simulink library "libbha_kinematic_tools"  (R2015b)
settings: Solver=FixedStepDiscrete  StartTime=0.0  StopTime=Inf  FixedStep=0.004  RelTol=1e-3
PostLoadFcn:
  | , if any(exist('dsrtsu_mdlpostloadfcn', 'file') == [2, 3, 6]), try dsrtsu_mdlpostloadfcn('Execute', bdroot); catch fprintf('Error in PostLoadFcn (dsrtsu_mdlpostloadfcn) for model "%s":\n %s\n', bdroot, lasterr); end, end,
undefined symbols (not defined in the file or in its folder): BHA
settings Model: DSRTSU_INTERNAL_RTI_VER=440  DSRTSU_INTERNAL_RTI_TYPE=rti1005  DSRTSU_INTERNAL_RTIFPGA=30  Creator=Falkenhahn  LastModifiedBy=Mayer
settings DataIOCC: SaveFormat=Array
settings OptimizationCC: BlockReduction=off  OptimizeBlockIOStorage=off  BufferReuse=off  GlobalBufferReuse=off  ExpressionFolding=off  LocalBlockOutputs=off
settings DebuggingCC: UnderspecifiedInitializationDetection=Classic  MergeDetectMultiDrivingBlocksExec=none  SolverPrmCheckMsg=warning
settings HardwareCC: ProdBitPerPointer=32  ProdLargestAtomicFloat=None  ProdEndianess=BigEndian  ProdWordSize=32  ProdHWDeviceType=Generic->Custom  TargetIntDivRoundTo=Zero  TargetEndianess=BigEndian  TargetHWDeviceType=Generic->Custom
settings RTWCC: SystemTargetFile=rti1007.tlc  MakeCommand=make_rti  TemplateMakefile=rti1007.tmf  Description=dSPACE DS1007 Hardware Platform
settings STFCustomTargetCC: ParMdlRefBuildCompliant=on  ConcurrentExecutionCompliant=off  MatFileLogging=on  SystemTargetFile=rti1007.tlc
settings GRTTargetCC: CompOptLevelCompliant=off  ConcurrentExecutionCompliant=off  GeneratePreprocessorConditionals=Disable all  CombineOutputUpdateFcns=off  GRTInterface=on  UseToolchainInfoCompliant=off  ExtModeMexFile=noextcomm
settings ConfigComp: CovModelRefEnable=Off

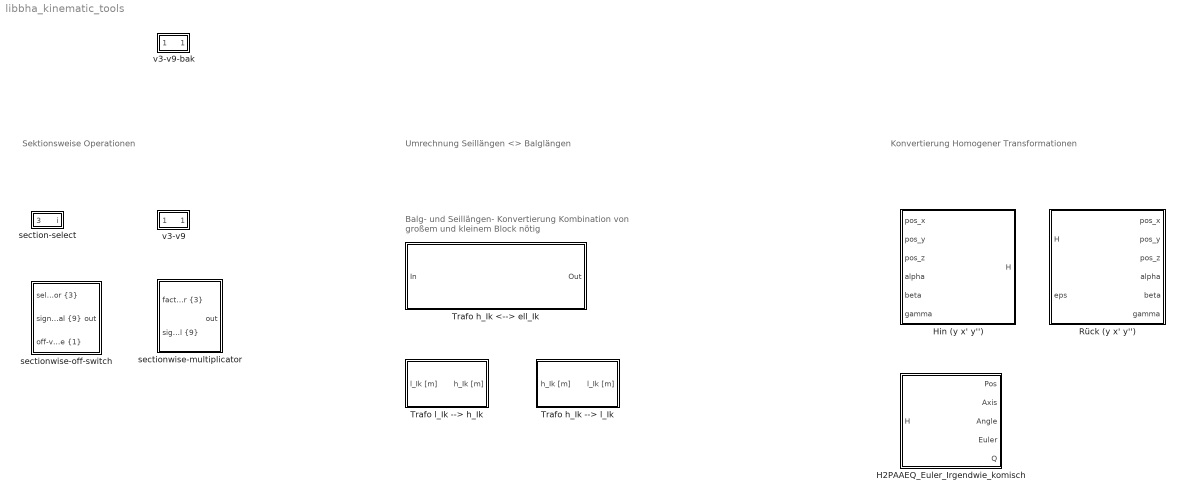
== system libbha_kinematic_tools ==
  note: Balg- und Seillängen- Konvertierung
      | Kombination von großem und kleinem Block nötig
  note: Konvertierung
      | Homogener Transformationen
  note: Umrechnung
      | Seillängen <> Balglängen
  note: Sektionsweise
      | Operationen
  H2PAAEQ_Euler_Irgendwie_komisch : MATLAB Function  TreatAsAtomicUnit=on
  Hin (y x' y'') : MATLAB Function  TreatAsAtomicUnit=on
  Rück (y x' y'') : MATLAB Function  TreatAsAtomicUnit=on
  Trafo h_Ik --> l_Ik : Subsystem  mask{ii=1 = gross}
      mask prompts: ii "Sektionsindex (ii)"
      settings: AttributesFormatString=Seilzughöhe > Seilzuglänge\nSektion = %<ii>
      mask TypeOptions ii: 1 = gross | 2 = mittel | 3 = klein
  Trafo h_Ik <--> ell_Ik : Subsystem  mask{inv=off, ii=1, m_i=BHA.Trunk.vc.num_segm, r_Si=BHA.Trunk.r_ms_i, r_Ai=BHA.Trunk.r_mb_i}
      mask prompts: inv "Transformationsrichtung (inv)"; ii "Sektionsindex (ii)"; m_i "Anzahl der Seilführungen, Segmente (m_i)"; r_Si "Radiale Abstände der Seilzugführungen von der Sektionsbiegelinie der i Sektionen (r_Si)"; r_Ai "Radiale Abstände der Aktoren von der Sektionsbiegelinie der i Sektionen (r_Ai)"
      mask help:
      | Berechnung der Hin- und Rücktransformation:
      | Balgbogenlänge ell_Ik <--> Seilzuglängen h_Ik
      |
      | Transformationsrichtung:
      |     - inv = disable:    h_Ik   --> ell_ik
      |     - inv = enable:     ell_Ik --> h_ik
      settings: AttributesFormatString=Seilzughöhe <> Balgbogenlänge\ninv = %<inv> | Sektion %<ii>
      mask Display: fprintf('inv = disable\n h_Ik -> ell_Ik \n\n inv = enable\n ell_Ik -> h_Ik')
  Trafo l_Ik --> h_Ik : Subsystem  mask{ii=1 = gross}
      mask prompts: ii "Sektionsindex (ii)"
      settings: AttributesFormatString=Seilzuglänge > Seilzughöhe\nSektion %<ii>
      mask TypeOptions ii: 1 = gross | 2 = mittel | 3 = klein
  section-select : Subsystem  mask(Sektionsauswahl){ii=1}
      mask prompts: ii "Sektion"
      mask help: wählt aus einem Parametersatz (Tripple) den der jew. Sektion aus
      settings: AttributesFormatString="in: 3  out: 1"
      mask Display: fprintf('S:%i',ii)
  sectionwise-multiplicator : Subsystem
  sectionwise-off-switch : Subsystem
  v3-v9 : Subsystem
  v3-v9-bak : Subsystem

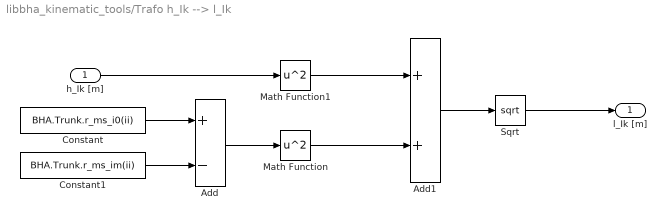
== system libbha_kinematic_tools/Trafo h_Ik --> l_Ik ==
  h_Ik [m] : Inport  PortDimensions=3
  Add : Sum  Inputs=+-
  Add1 : Sum
  Constant : Constant  Value=BHA.Trunk.r_ms_i0(ii)
  Constant1 : Constant  Value=BHA.Trunk.r_ms_im(ii)
  Math Function : Math  Operator=square  SaturateOnIntegerOverflow=on
  Math Function1 : Math  Operator=square  SaturateOnIntegerOverflow=on
  Sqrt : Sqrt  SaturateOnIntegerOverflow=on
  l_Ik [m] : Outport  PortDimensions=3
  wires:
  Constant/1 -> Add/1
  Constant1/1 -> Add/2
  Add/1 -> Math Function/1
  Math Function/1 -> Add1/2
  h_Ik [m]/1 -> Math Function1/1
  Math Function1/1 -> Add1/1
  Add1/1 -> Sqrt/1
  Sqrt/1 -> l_Ik [m]/1

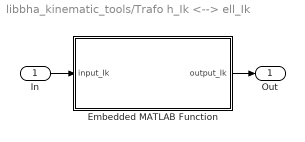
== system libbha_kinematic_tools/Trafo h_Ik <--> ell_Ik ==
  In : Inport  PortDimensions=[3,1]
  Embedded MATLAB Function : MATLAB Function  TreatAsAtomicUnit=on
  Out : Outport  PortDimensions=[3,1]
  wires:
  In/1 -> Embedded MATLAB Function/1(input_Ik)
  Embedded MATLAB Function/1(output_Ik) -> Out/1

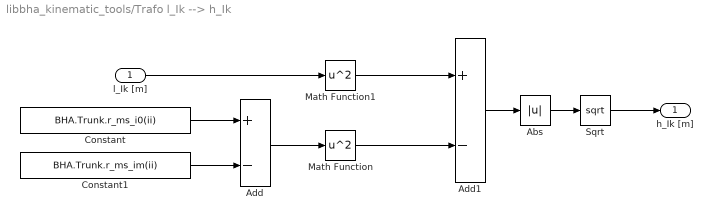
== system libbha_kinematic_tools/Trafo l_Ik --> h_Ik ==
  l_Ik [m] : Inport  PortDimensions=3
  Abs : Abs
  Add : Sum  Inputs=+-
  Add1 : Sum  Inputs=+-
  Constant : Constant  Value=BHA.Trunk.r_ms_i0(ii)
  Constant1 : Constant  Value=BHA.Trunk.r_ms_im(ii)
  Math Function : Math  Operator=square  SaturateOnIntegerOverflow=on
  Math Function1 : Math  Operator=square  SaturateOnIntegerOverflow=on
  Sqrt : Sqrt  SaturateOnIntegerOverflow=on
  h_Ik [m] : Outport  PortDimensions=3
  wires:
  Abs/1 -> Sqrt/1
  Sqrt/1 -> h_Ik [m]/1
  Add1/1 -> Abs/1
  Math Function1/1 -> Add1/1
  l_Ik [m]/1 -> Math Function1/1
  Math Function/1 -> Add1/2
  Add/1 -> Math Function/1
  Constant1/1 -> Add/2
  Constant/1 -> Add/1

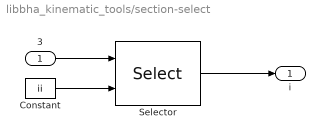
== system libbha_kinematic_tools/section-select ==
  3 : Inport
  Constant : Constant  Value=ii
  Selector : Selector  InputPortWidth=3  IndexOptions=Index vector (port)  Indices=[1 3]  OutputSizes=1
  i : Outport
  wires:
  3/1 -> Selector/1
  Selector/1 -> i/1
  Constant/1 -> Selector/2

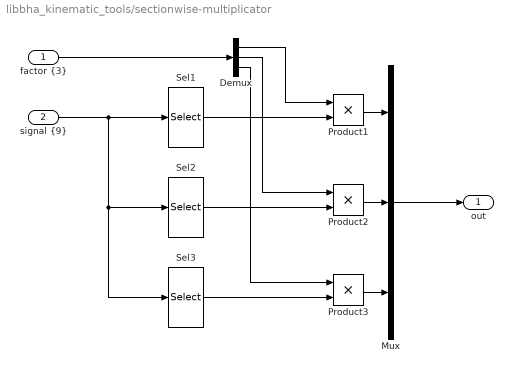
== system libbha_kinematic_tools/sectionwise-multiplicator ==
  "factor {3}" : Inport
  "signal {9}" : Inport  Port=2
  Demux : Demux  Outputs=3
  Mux : Mux  Inputs=3
  Product1 : Product  RndMeth=Zero
  Product2 : Product  RndMeth=Zero
  Product3 : Product  RndMeth=Zero
  Sel1 : Selector  InputPortWidth=9  IndexOptions=Index vector (dialog)  Indices=[1 2 3]  OutputSizes=1
  Sel2 : Selector  InputPortWidth=9  IndexOptions=Index vector (dialog)  Indices=[4 5 6]  OutputSizes=1
  Sel3 : Selector  InputPortWidth=9  IndexOptions=Index vector (dialog)  Indices=[7 8 9]  OutputSizes=1
  out : Outport
  wires:
  Demux/3 -> Product3/1
  Demux/2 -> Product2/1
  Demux/1 -> Product1/1
  Sel1/1 -> Product1/2
  Mux/1 -> out/1
  "signal {9}"/1 -> Sel3/1, Sel2/1, Sel1/1
  Product2/1 -> Mux/2
  Product3/1 -> Mux/3
  Sel3/1 -> Product3/2
  Product1/1 -> Mux/1
  Sel2/1 -> Product2/2
  "factor {3}"/1 -> Demux/1

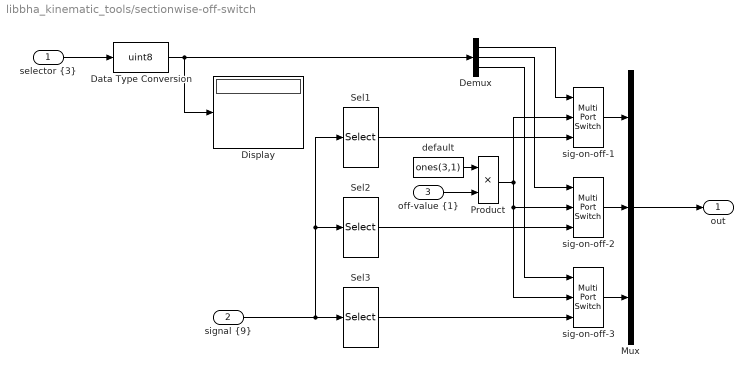
== system libbha_kinematic_tools/sectionwise-off-switch ==
  "selector {3}" : Inport
  "signal {9}" : Inport  Port=2
  "off-value {1}" : Inport  Port=3
  Data Type Conversion : DataTypeConversion  OutDataTypeStr=uint8
  Demux : Demux  Outputs=3
  Display : Display
  Mux : Mux  Inputs=3
  Product : Product  RndMeth=Zero
  Sel1 : Selector  InputPortWidth=9  IndexOptions=Index vector (dialog)  Indices=[1 2 3]  OutputSizes=1
  Sel2 : Selector  InputPortWidth=9  IndexOptions=Index vector (dialog)  Indices=[4 5 6]  OutputSizes=1
  Sel3 : Selector  InputPortWidth=9  IndexOptions=Index vector (dialog)  Indices=[7 8 9]  OutputSizes=1
  default : Constant  Value=ones(3,1)
  sig-on-off-1 : MultiPortSwitch  DataPortOrder=Zero-based contiguous  Inputs=2  DiagnosticForDefault=None
  sig-on-off-2 : MultiPortSwitch  DataPortOrder=Zero-based contiguous  Inputs=2  DiagnosticForDefault=None
  sig-on-off-3 : MultiPortSwitch  DataPortOrder=Zero-based contiguous  Inputs=2  DiagnosticForDefault=None
  out : Outport
  wires:
  Sel1/1 -> sig-on-off-1/3
  Sel2/1 -> sig-on-off-2/3
  Sel3/1 -> sig-on-off-3/3
  Data Type Conversion/1 -> Demux/1, Display/1
  default/1 -> Product/1
  "off-value {1}"/1 -> Product/2
  Demux/3 -> sig-on-off-3/1
  Demux/2 -> sig-on-off-2/1
  Product/1 -> sig-on-off-2/2, sig-on-off-3/2, sig-on-off-1/2
  Demux/1 -> sig-on-off-1/1
  "selector {3}"/1 -> Data Type Conversion/1
  sig-on-off-1/1 -> Mux/1
  sig-on-off-3/1 -> Mux/3
  sig-on-off-2/1 -> Mux/2
  "signal {9}"/1 -> Sel3/1, Sel2/1, Sel1/1
  Mux/1 -> out/1

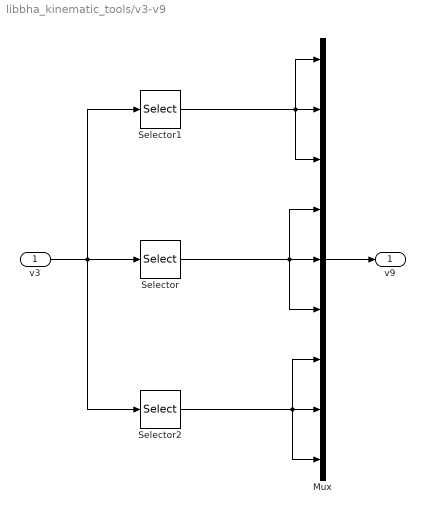
== system libbha_kinematic_tools/v3-v9 ==
  v3 : Inport
  Mux : Mux  Inputs=9
  Selector : Selector  InputPortWidth=3  IndexOptions=Index vector (dialog)  Indices=[2]  OutputSizes=1
  Selector1 : Selector  InputPortWidth=3  IndexOptions=Index vector (dialog)  Indices=[1 ]  OutputSizes=1
  Selector2 : Selector  InputPortWidth=3  IndexOptions=Index vector (dialog)  Indices=[3]  OutputSizes=1
  v9 : Outport
  wires:
  Selector/1 -> Mux/6, Mux/4, Mux/5
  Selector1/1 -> Mux/3, Mux/1, Mux/2
  Selector2/1 -> Mux/9, Mux/7, Mux/8
  Mux/1 -> v9/1
  v3/1 -> Selector2/1, Selector1/1, Selector/1

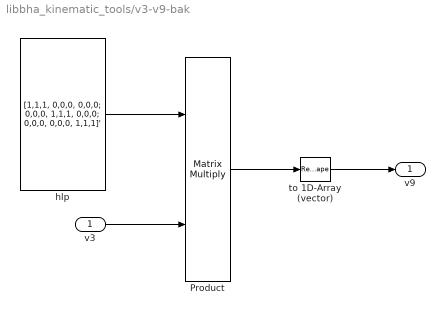
== system libbha_kinematic_tools/v3-v9-bak ==
  v3 : Inport
  Product : Product  Multiplication=Matrix(*)  RndMeth=Zero
  hlp : Constant  Value=[1,1,1, 0,0,0, 0,0,0; 0,0,0, 1,1,1, 0,0,0; 0,0,0, 0,0,0, 1,1,1]'
  to 1D-Array (vector) : Reshape
  v9 : Outport
  wires:
  v3/1 -> Product/2
  hlp/1 -> Product/1
  Product/1 -> to 1D-Array (vector)/1
  to 1D-Array (vector)/1 -> v9/1

== matlab function libbha_kinematic_tools/Hin (y x' y'') ==
  data: pos_x input; pos_y input; pos_z input; alpha input; H output; beta input; gamma input
function H = EulerYXY2H(pos_x, pos_y, pos_z, alpha, beta, gamma)
%#codegen

%H = [   cos(beta)*cos(gamma)    cos(alpha)*sin(gamma)+sin(alpha)*sin(beta)*cos(gamma)   sin(alpha)*sin(gamma)-cos(alpha)*sin(beta)*cos(gamma)   2; ...
%        -cos(beta)*sin(gamma)   cos(alpha)*cos(gamma)-sin(alpha)*sin(beta)*sin(gamma)   sin(alpha)*cos(gamma)+cos(alpha)*sin(beta)*sin(gamma)   3; ...
%        sin(beta)               -sin(alpha)*cos(beta)                                   cos(alpha)*cos(beta)                                    4; ...
%        0                                                       0                                                       0                       1 ];

% Drehung um y
A1 = [  cos(alpha)  0   sin(alpha)  ;
        0           1   0           ;
        -sin(alpha) 0   cos(alpha)  ];


% Drehung um x
A2 = [  1   0           0           ;
        0   cos(beta)   -sin(beta)  ;
        0   sin(beta)   cos(beta)   ];

% Drehung um y
A3 = [  cos(gamma)  0   sin(gamma)  ;
        0           1   0           ;
        -sin(gamma) 0   cos(gamma)  ];


H = [ A3*A2*A1 , [pos_x;pos_y;pos_z]; [0, 0, 0, 1]];

== matlab function libbha_kinematic_tools/Rück (y x' y'') ==
  data: pos_x output; pos_y output; pos_z output; alpha output; H input; beta output; gamma output; eps input
function [pos_x, pos_y, pos_z, alpha, beta, gamma] = H2EulerYXY(H, eps)
    %% Position
    
    pos_x = H(1,4);
    pos_y = H(2,4);
    pos_z = H(3,4);


    %% Winkel
    % 1. Drehung um y
    % 2. Drehung um x'
    % 3. Drehung um y''
    
    cb = H(2,2);

    if abs(cb) > eps 
        beta = acos(real(cb));
        
        if abs(sin(beta)) > eps % allgemein
            alpha = atan2( H(2,1)/sin(beta), -H(2,3)/sin(beta) );
            gamma = atan2( H(1,2)/sin(beta),  H(3,2)/sin(beta) );
            
        else % beta = 0 | pi | 2 pi ...
            gamma = 0.0; % Zweite Drehung sorgt für Übereinstimmung/Singularität zwischen Drehung 1 (alpha) und Drehung 3 (gamma). Drehung 3 wird zu 0 gesetzt und alles auf eine resultierende Drehung 1 umgerechnet.
            
            if cb > 0 % beta = 0 | 2 pi | ...
                beta = 0.0;
                alpha = ( acos(H(1,1)) + acos(H(3,3)) + asin(H(1,3)) + asin(-H(3,1)) )/4;
            else % beta = pi | 3 pi ...
                beta = pi;
                
                if H(3,1)+H(1,3) > 0 % alpha - gamma > 0
                    alpha =  (acos(H(1,1))-acos(H(3,3)))/2;
                else
                    alpha = -(acos(H(1,1))-acos(H(3,3)))/2;
                end

            end          
        end
    else % cos(beta)=0: beta = 0.5 pi | 1.5 pi | 3.5 pi ...
        % sin(beta)=1, beta = 0.5 pi | 3.5 pi ...
        alphap = atan2( H(2,1), -H(2,3) );
        gammap = atan2( H(1,2),  H(3,2) );
        betap = pi/2;
        
        % sin(beta)=-1, beta = 1.5 pi | 4.5 pi ...
        alpham = atan2( -H(2,1),  H(2,3) );
        gammam = atan2( -H(1,2), -H(3,2) );
        betam = -pi/2;

        % Vergleich Fehler
        sbp = abs( sin(gammap)*sin(betap)-H(1,2))+abs( sin(betap)*sin(alphap)-H(2,1))+abs(-sin(betap)*cos(alphap)-H(2,3))+abs( cos(gammap)*sin(betap)-H(3,2));
        sbn = abs( sin(gammam)*sin(betam)-H(1,2))+abs( sin(betam)*sin(alpham)-H(2,1))+abs(-sin(betam)*cos(alpham)-H(2,3))+abs( cos(gammam)*sin(betam)-H(3,2));
        
        if sbp < sbn
            alpha = alphap;
            beta = betap;
            gamma = gammap;
        else
            alpha = alpham;
            beta = betam;
            gamma = gammam;
        end
    end
    
end

== matlab function libbha_kinematic_tools/H2PAAEQ_Euler_Irgendwie_komisch ==
  data: H input size=[4,4]; Pos output size=[1 3]; Axis output size=[1 3]; Angle output size=1; Euler output size=[1 3]; Q output size=4
function [Pos, Axis, Angle, Euler, Q] = fcn(H)
    % Input:    
    % - Homogene Transformationsmatrix H
    % Output:
    % - Position Pos (x y z)
    % - Drehachse Axis
    % - Drehwinkel Angle
    % - Eulerwinkel Euler (heading:rot(y), attitude:rot(z), bank:rot(x))
    % - Quaternionen Q

    %% Position
    Pos     = H(1:3, 4)';
    x = Pos(1);
    y = Pos(2);
    z = Pos(3);

    %% Achse und Drehwinkel
    Angle   = acos((H(1,1)+H(2,2)+H(3,3)-1)/2);

    if abs(sin(Angle)) < 1e-6
        if abs(1-cos(Angle)) < 1e-6
            Axis = [1,0,0];
        else
            abs_x = sqrt((H(1,1)+1)/2);
            abs_y = sqrt((H(2,2)+1)/2);
            abs_z = sqrt((H(3,3)+1)/2);

            Axis = [abs_x,...
                    abs_y * sign(H(1,2)),...
                    abs_z * sign(H(1,3))];
        end
    else
        Axis = 1/(2*sin(Angle))*[H(3,2)-H(2,3),...
                                 H(1,3)-H(3,1),...
                                 H(2,1)-H(1,2)];
    end

    %% Eulerwinkel

    % 	heading = atan2(y * sin(angle)- x * z * (1 - cos(angle)) , 1 - (y^2 + z^2 ) * (1 - cos(angle)));
    % 	attitude = asin(x * y * (1 - cos(angle)) + z * sin(angle));
    % 	bank = atan2(x * sin(angle)-y * z * (1 - cos(angle)) , 1 - (x^2 + z^2) * (1 - cos(angle)));
    s=sin(Angle);
    t=1-cos(Angle);
    
    %  if axis is not already normalised then uncomment this
	% magnitude = sqrt(x*x + y*y + z*z);
	% if (magnitude==0) throw error;
	% x /= magnitude;
	% y /= magnitude;
	% z /= magnitude;
    if ((x*y*t + z*s) > 0.998)  % north pole singularity detected
		heading = 2*bha_atan2(x*sin(Angle/2),cos(Angle/2));
		attitude = pi/2;
		bank = 0;
	elseif ((x*y*t + z*s) < -0.998)  % south pole singularity detected
		heading = -2*bha_atan2(x*sin(Angle/2),cos(Angle/2));
		attitude = -pi/2;
		bank = 0;
	else
        heading = bha_atan2(y * s- x * z * t , 1 - (y*y+ z*z ) * t);
        attitude = asin(x * y * t + z * s) ;
        bank = bha_atan2(x * s - y * z * t , 1 - (x*x + z*z) * t);
    end

    % Euler = [heading attitude bank];
    Euler = [bank heading attitude];
    
    %% Quaternionen
    
    cth  =   cos(bank/2);
    sth  =   sin(bank/2);

    cph  =   cos(heading/2);
    sph  =   sin(heading/2);

    cps  =   cos(attitude/2);
    sps  =   sin(attitude/2);

    Q    = [ cth*cph*cps+sth*sph*sps; ...
             sth*cph*cps-cth*sph*sps; ...
             cth*sph*cps+sth*cph*sps; ...
             cth*cph*sps-sth*sph*cps ]; 
    
end


function y = bha_atan2(u1, u2)
    % Spezielle Arcustangensfunktion, da der PLC-Coder atan2 nicht
    % übersetzen kann. Muss in untergeordnete EmbeddedMatlabFunctions
    % DIREKT eingebunden werden (copy/paste)

	%#codegen

% 	if u2 > 0
% 		y = atan(u1/u2);
% 	elseif u2 < 0
% 		if u1 >= 0
% 			y = atan(u1/u2) + pi;
% 		else 
% 			y = atan(u1/u2) - pi;
% 		end
% 	else
% 		if u1 > 0.0
% 			y = pi/2;
% 		elseif u1 < 0.0
% 			y = -pi/2;
% 		else 
% 			y = 0.0;
% 		end
% 	end

y = atan2(u1,u2);
	
end

== matlab function libbha_kinematic_tools/Trafo h_Ik <--> ell_Ik/Embedded MATLAB Function ==
  data: input_Ik input size=[3,1]; inv parameter; output_Ik output size=[3,1]; ii parameter; m_i parameter; r_Si parameter; r_Ai parameter
function output_Ik = fcn(input_Ik, inv, ii, m_i, r_Si, r_Ai)
% XXXXXXXXXXXXXXXXXXXXXXXXXXXXXXXXXXXXXXXXXXXXXXXXXXXXXXXXXXXXXXXXXXXXXXXXX
% Funktion zur Berechnung der Hin- und Rücktransformation
% Balgbogenlänge ell_Ik <--> Seilzuglängen h_Ik
%
% Modell Seilzughöhen: Constant Curvature Cable-Driven
% Modell Balgaktor: Constant Curvature Continuum
%
% inv = disable
%   Input:
%       - input_Ik = h_Ik       [3x1]   Seilzughöhen (= Seilzuglängen korrigiert um Konizität des Aktors)
%   Output:
%       - output_Ik = ell_Ik    [3x1]   Aktorbogenlängen
%
% inv = enable
%   Input:
%       - input_Ik = ell_Ik     [3x1]   Aktorbogenlängen
%   Output:
%       - output_Ik = h_Ik      [3x1]   Seilzughöhen (= Seilzuglängen korrigiert um Konizität des Aktors)
%
% Parameter:
%   - inv       [1x1]   Richtung der Transformation
%   - ii        [1x1]   Sektionsindex
%   - m_i       [nx1]   Anzahl der Seilführungen (Segmente) der i Sektionen 
%   - r_Si      [nx1]   Radiale Abstände der Seilzugführungen von der Sektionsbiegelinie der i Sektionen 
%   - r_Ai      [nx1]   Radiale Abstände der Aktoren von der Sektionsbiegelinie der i Sektionen 

    if inv == 0
        k_I         = f_specific_I_cable(input_Ik, m_i(ii), r_Si(ii));
        output_Ik   = inv_f_specific_I_continuum(k_I, r_Ai(ii));
    else
        k_I         = f_specific_I_continuum(input_Ik, r_Ai(ii));
        output_Ik   = inv_f_specific_I_cable(k_I, m_i(ii), r_Si(ii));
    end

end

% XXXXXXXXXXXXXXXXXXXXXXXXXXXXXX CONTINUUM XXXXXXXXXXXXXXXXXXXXXXXXXXXXXXXX
function k_I = f_specific_I_continuum(ell_Ik, r_I)

% Berechnung der Transformation
% Aktorbogenlängen ell_Ik --> Konfigurationszustand [phi_I, kappa_I, ell_I]  
% einer einzelnen Sektion gemäß der Abbildung:
% k_I = f_specific_I_continuum(ell_Ik)
% 
% Input:
%   ell_Ik  [3x1]   Aktorbogenlängen (kontinuierlich biegender Aktor)
%
% Output:
%   k_I     [3x1]   Konfigurationszustand (phi_I, kappa_I, ell_I)
%
% Parameter:
%   r_I     [1x1]   Radialer Abstand der Aktoren

    % Singularität für wurzel=0 ! -> Definition des singulären Gebiets
    eps     = 1e-6;
    wurzel = sqrt(max([0, ell_Ik(1,1)^2 + ell_Ik(2,1)^2 + ell_Ik(3,1)^2 - ell_Ik(1,1)*ell_Ik(2,1) - ell_Ik(1,1)*ell_Ik(3,1) - ell_Ik(2,1)*ell_Ik(3,1)]));
    
    if wurzel < eps
        phi_I  = bha_atan2(sqrt(3)*(ell_Ik(3,1)-ell_Ik(2,1)), ell_Ik(2,1)+ell_Ik(3,1)-2*ell_Ik(1,1));
        kappa_I= 0;
        ell_I  = (ell_Ik(1,1)+ell_Ik(2,1)+ell_Ik(3,1))/3;    
    else
        phi_I  = bha_atan2(sqrt(3)*(ell_Ik(3,1)-ell_Ik(2,1)), ell_Ik(2,1)+ell_Ik(3,1)-2*ell_Ik(1,1));
        kappa_I= 2*wurzel / (r_I*(ell_Ik(1,1)+ell_Ik(2,1)+ell_Ik(3,1)));
        ell_I  = (ell_Ik(1,1)+ell_Ik(2,1)+ell_Ik(3,1))/3;
    end
    
    k_I    = [phi_I; kappa_I; ell_I];
end

function ell_Ik = inv_f_specific_I_continuum(k_I, r_I)
% Berechnung der inversen Transformation
% Aktorbogenlängen ell_Ik <-- Konfigurationszustand [phi_I, kappa_I, ell_I]  
% einer einzelnen Sektion gemäß der Abbildung:
% ell_Ik = inv_f_specific_I_continuum(k_I)
% 
% Input:
%   k_I     [3x1]   Konfigurationszustand (phi_I, kappa_I, ell_I)
%
% Output:
%   ell_Ik  [3x1]   Aktorbogenlängen (kontinuierlich biegender Aktor)
%
% Parameter:
%   r_I     [1x1]   Radialer Abstand der Aktoren

    phi_I   = k_I(1);
    kappa_I = k_I(2);
    ell_I   = k_I(3);
    
    ell_Ik = ell_I*ones(3,1) - kappa_I*ell_I*r_I*cos(2*[0;1;2]*pi./3 - phi_I*ones(3,1));
end

% XXXXXXXXXXXXXXXXXXXXXXXXXXX CABLE XXXXXXXXXXXXXXXXXXXXXXXXXXXXXXXXXXXXXXX
function k_I = f_specific_I_cable(h_Ik, m_I, r_I)

% Berechnung der Transformation
% Seilzughöhen h_Ik --> Konfigurationszustand [phi_I, kappa_I, ell_I]  
% einer einzelnen Sektion gemäß der Abbildung:
% k_I = f_specific_I_cable(h_Ik)
% 
% Input:
%   h_Ik    [3x1]   Seizuglängen (Seilzugaktor)
%
% Output:
%   k_I     [3x1]   Konfigurationszustand (phi_I, kappa_I, ell_I)
%
% Parameter:
%   r_I     [1x1]   Radialer Abstand der Seilzüge

    % Singularität für wurzel=0 ! -> Definition des singulären Gebiets
    eps     = 1e-6;
    wurzel = sqrt(max([0, h_Ik(1,1)^2 + h_Ik(2,1)^2 + h_Ik(3,1)^2 - h_Ik(1,1)*h_Ik(2,1) - h_Ik(1,1)*h_Ik(3,1) - h_Ik(2,1)*h_Ik(3,1)]));
    
    if wurzel < eps
        phi_I  = bha_atan2(sqrt(3)*(h_Ik(3,1)-h_Ik(2,1)), h_Ik(2,1)+h_Ik(3,1)-2*h_Ik(1,1));
        kappa_I= 0;
        ell_I  = (h_Ik(1,1)+h_Ik(2,1)+h_Ik(3,1))/3;
    else
        phi_I  = bha_atan2(sqrt(3)*(h_Ik(3,1)-h_Ik(2,1)), h_Ik(2,1)+h_Ik(3,1)-2*h_Ik(1,1));
        kappa_I= 2*wurzel / (r_I*(h_Ik(1,1)+h_Ik(2,1)+h_Ik(3,1)));
        ell_I  = 2*m_I/kappa_I * asin(wurzel/(3*r_I*m_I));
    end
    
    k_I    = [phi_I; kappa_I; ell_I];
end

function h_Ik = inv_f_specific_I_cable(k_I, m_I, r_I)
% Inverse Berechnung der Transformation
% Seilzughöhen h_Ik <-- Konfigurationszustand [phi_I, kappa_I, ell_I]  
% einer einzelnen Sektion gemäß der Abbildung:
% h_Ik = inv_f_specific_I_cable(k_I)
% 
% Input:
%   k_I     [3x1]   Konfigurationszustand (phi_I, kappa_I, ell_I)
%
% Output:
%   h_Ik    [3x1]   Seizuglängen (Seilzugaktor)
%
% Parameter:
%   r_I     [1x1]   Radialer Abstand der Seilzüge

    phi_I   = k_I(1);
    kappa_I = k_I(2);
    ell_I   = k_I(3);
    
    % Singularität für kappa_I=0 ! -> Definition des singulären Gebiets
    eps = 1e-7;
    
    if kappa_I<eps
        h_Ik = ell_I*ones(3,1);
    else
        h_Ik = 2*m_I*sin(kappa_I*ell_I/2/m_I)*(1/kappa_I*ones(3,1) - r_I*cos(2*[0;1;2]*pi./3 - phi_I*ones(3,1)));
    end
end


function y = bha_atan2(u1, u2)
% Eigene Arcustangens2funktion, da der PLC-Coder atan2 nicht
% übersetzen kann.

	if u2 > 0
		y = atan(u1/u2);
	elseif u2 < 0
		if u1 >= 0
			y = atan(u1/u2) + pi;
		else 
			y = atan(u1/u2) - pi;
		end
	else
		if u1 > 0.0
			y = pi/2;
		elseif u1 < 0.0
			y = -pi/2;
		else 
			y = 0.0;
		end
	end
	
end
